simulink model "QEI_simulink_model"  (R2018a)
settings: Solver=VariableStepAuto  StartTime=0.0  StopTime=10.0  RelTol=1e-3
values from neighbouring files (symbols this model uses):
  b = tan(pi/M/2)    [QEI.m]
libraries: simulink x1
settings Model: Creator=Felipe  LastModifiedBy=Felipe

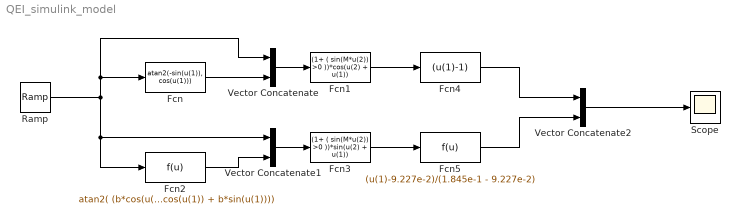
== system QEI_simulink_model ==
  Fcn : Fcn  Expr=atan2(-sin(u(1)), cos(u(1)))
  Fcn1 : Fcn  Expr=(1+ ( sin(M*u(2)) >0 ))*cos(u(2) + u(1))
  Fcn2 : Fcn  Expr=atan2( (b*cos(u(1)) - sin(u(1))), (cos(u(1)) + b*sin(u(1))))
  Fcn3 : Fcn  Expr=(1+ ( sin(M*u(2)) >0 ))*sin(u(2) + u(1))
  Fcn4 : Fcn  Expr=(u(1)-1)
  Fcn5 : Fcn  Expr=(u(1)-9.227e-2)/(1.845e-1 - 9.227e-2)
  Ramp : simulink/Sources/Ramp  slope=0.2  start=0  InitialOutput=0
  Scope : Scope
  Vector Concatenate : Concatenate
  Vector Concatenate1 : Concatenate
  Vector Concatenate2 : Concatenate
  wires:
  Fcn1/1 -> Fcn4/1
  Vector Concatenate/1 -> Fcn1/1
  Fcn/1 -> Vector Concatenate/2
  Vector Concatenate1/1 -> Fcn3/1
  Fcn2/1 -> Vector Concatenate1/2
  Ramp/1 -> Vector Concatenate/1, Fcn/1, Fcn2/1, Vector Concatenate1/1
  Vector Concatenate2/1 -> Scope/1
  Fcn4/1 -> Vector Concatenate2/1
  Fcn3/1 -> Fcn5/1
  Fcn5/1 -> Vector Concatenate2/2
